simulink library "EU_Tapping_Cycle"  (R2018b)
settings: Solver=ode45  StartTime=0.0  StopTime=10.0  RelTol=1e-3  EnableMultiTasking=on
libraries: carnot x1
settings Model: Creator=lena.frank  LastModifiedBy=P41573
settings DataIOCC: LimitDataPoints=on  SaveFormat=Array  SignalLoggingSaveFormat=ModelDataLogs
settings OptimizationCC: ExpressionDepthLimit=2147483647  LifeSpan=inf
settings DebuggingCC: UnderspecifiedInitializationDetection=Classic  MergeDetectMultiDrivingBlocksExec=none  SolverPrmCheckMsg=warning  FcnCallInpInsideContextMsg=warning  StateNameClashWarn=warning  SFUnexpectedBacktrackingDiag=warning  SFNoUnconditionalDefaultTransitionDiag=warning  SFExecutionAtInitializationDiag=none
settings HardwareCC: ProdBitPerPointer=32  ProdBitPerSizeT=32  ProdBitPerPtrDiffT=32  ProdLargestAtomicFloat=None  ProdIntDivRoundTo=Undefined  ProdEndianess=Unspecified  ProdWordSize=32  ProdHWDeviceType=32-bit Generic
settings ModelReferenceCC: PropagateSignalLabelsOutOfModel=off
settings SFSimCC: SimUseLocalCustomCode=off
settings RTWCC: RTWUseLocalCustomCode=off
settings CodeAppCC: StateflowObjectComments=on
settings GRTTargetCC: TargetLangStandard=C89/C90 (ANSI)  GeneratePreprocessorConditionals=Disable all  CombineOutputUpdateFcns=off  GRTInterface=on
settings ConfigComp: CovMetricSettings=dw  CovHtmlReporting=on  CovSaveCumulativeToWorkspaceVar=on  CovSaveSingleToWorkspaceVar=on  CovExternalEMLEnable=off

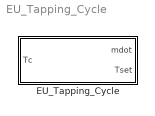
== system EU_Tapping_Cycle ==
  EU_Tapping_Cycle : Subsystem  mask(European tapping cycles){eu_tap=M, dTbias=0}
      mask prompts: eu_tap "EU Tapping Cycle Number"; dTbias "Bias on setpoint temperature in K"
      mask help:
      | European tapping cycles developped according to Mandate 324 and used in various standards for energy labelling and eco design of hot water heaters and hot water storage tanks.
      | The check of mean temperature Tm and peak temperature Tp must be done in a post treatment of the simulation data. A bias on the setpoint temperature can be defined. This assures that the tapping temperature is above the (minimum) setpoint given by the tapping cycle.
      mask init:
      | [times, energies, dT_set, mdot] = ...
      |     CarnotCallbacks_EU_Tapping_Cycle(eu_tap, dTbias);
      mask Help: web(fullfile(path_carnot('help'),'EuTappingCycle.html'),'-helpbrowser')
      mask TypeOptions eu_tap: 3XS | XXS | XS | S | M | L | XL | XXL | 3XL | 4XL
      mask Display: disp('EU tapping\n from 3XS\nto 4XL')

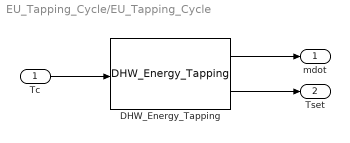
== system EU_Tapping_Cycle/EU_Tapping_Cycle ==
  Tc : Inport
  DHW_Energy_Tapping : carnot/Load/Hot_Water_Tapping/DHW_Energy_Tapping  mdot_nom=1  times=times  energies=energies  dT_set=dT_set  coeffs=mdot
      settings: SourceProductName=Carnot
  mdot : Outport
  Tset : Outport  Port=2
  wires:
  Tc/1 -> DHW_Energy_Tapping/1
  DHW_Energy_Tapping/2 -> Tset/1
  DHW_Energy_Tapping/1 -> mdot/1
